simulink model "Propeller"  (R2021a)
settings: Solver=VariableStepAuto  StartTime=0.0  StopTime=10.0  RelTol=1e-3
values from neighbouring files (symbols this model uses):
  param = struct()    [parameters.m]
libraries: vrlib x1
settings Model: Creator=PC  LastModifiedBy=PC

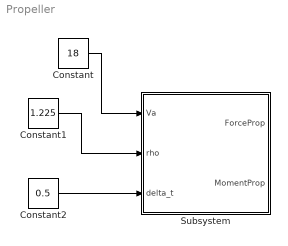
== system Propeller ==
  Constant : Constant  Value=18
  Constant1 : Constant  Value=1.225
  Constant2 : Constant  Value=0.5
  Subsystem : Subsystem
  wires:
  Constant/1 -> Subsystem/1(Va)
  Constant1/1 -> Subsystem/2(rho)
  Constant2/1 -> Subsystem/3(delta_t)

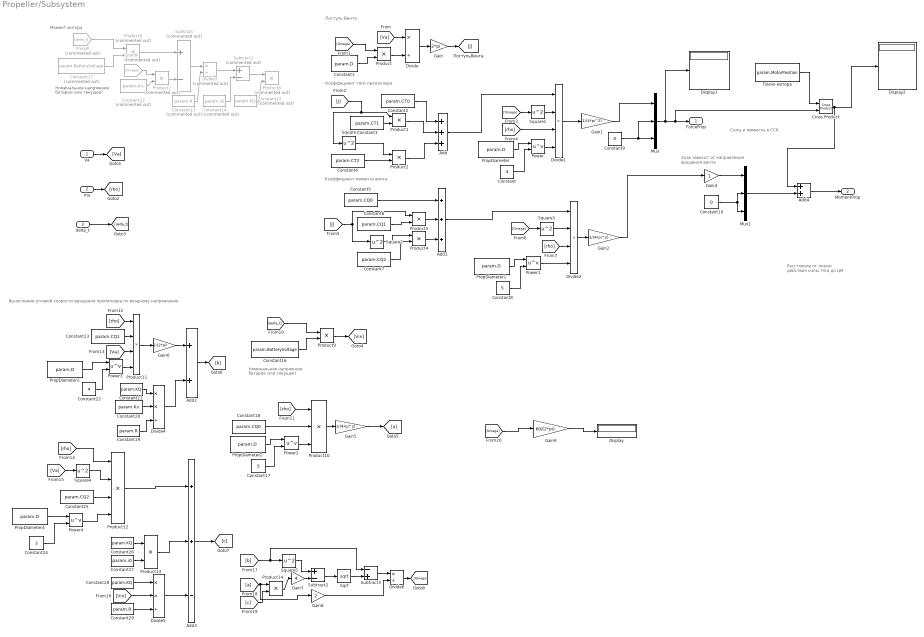
== system Propeller/Subsystem ==
  note: Вычисление угловой скорости вращения пропеллера по входному напряжению
  note: Момент мотора
  note: Номинальное напряжние
      | батарии или текущее?
  note: Знак зависит от направления
      | вращения винта
  note: Силы и моменты в ССК
  note: Расстояние от линии
      | действия силы тяги до ЦМ
  note: Коэффициент момента винта
  note: Коэффициент тяги пропеллера
  note: Поступь Винта
  note: Номинальное напряжние
      | батарии или текущее?
  Va : Inport
  rho : Inport  Port=2
  delta_t : Inport  Port=3
  Add : Sum  Inputs=+++
  Add1 : Sum  Inputs=+++
  Add2 : Sum
  Add3 : Sum  Inputs=++-
  Add4 : Sum
  Constant : Constant  Value=4
  Constant1 : Constant  Value=param.D
  Constant10 : Constant  Value=0
  Constant11 : Constant  Commented=on  Value=param.BatteryVoltage
  Constant12 : Constant  Commented=on  Value=param.Kv
  Constant13 : Constant  Commented=on  Value=param.R
  Constant14 : Constant  Commented=on  Value=param.i0
  Constant15 : Constant  Commented=on  Value=param.KQ
  Constant16 : Constant  Value=param.BatteryVoltage
  Constant17 : Constant  Value=5
  Constant18 : Constant  Value=param.CQ0
  Constant19 : Constant  Value=param.R
  Constant2 : Constant  Value=param.CT0
  Constant20 : Constant  Value=param.Kv
  Constant21 : Constant  Value=param.KQ
  Constant22 : Constant  Value=4
  Constant23 : Constant  Value=param.CQ1
  Constant24 : Constant  Value=3
  Constant25 : Constant  Value=param.CQ2
  Constant26 : Constant  Value=param.KQ
  Constant27 : Constant  Value=param.i0
  Constant28 : Constant  Value=param.KQ
  Constant29 : Constant  Value=param.R
  Constant3 : Constant  Value=param.CT1
  Constant4 : Constant  Value=param.CT2
  Constant5 : Constant  Value=param.CQ0
  Constant6 : Constant  Value=param.CQ1
  Constant7 : Constant  Value=param.CQ2
  Constant8 : Constant  Value=5
  Constant9 : Constant  Value=0
  Cross Product : vrlib/Utilities/Cross Product
  Display : Display
  Display1 : Display
  Display2 : Display
  Divide : Product  Inputs=*/
  Divide1 : Product  Inputs=****
  Divide2 : Product  Inputs=****
  Divide3 : Product  Commented=on  Inputs=*/
  Divide4 : Product  Inputs=**/
  Divide5 : Product  Inputs=**/
  Divide6 : Product  Inputs=*/
  From8 : From  Commented=on  GotoTag=delta_t
  From9 : From  Commented=on  GotoTag=Omega
  Gain : Gain  Gain=2*pi
  Gain1 : Gain  Gain=1/(4*pi^2)
  Gain2 : Gain  Gain=1/(4*pi^2)
  Gain4 : Gain
  Gain5 : Gain  Gain=1/(4*pi^2)
  Gain6 : Gain  Gain=1/(2*pi)
  Gain7 : Gain  Gain=4
  Gain8 : Gain  Gain=2
  Gain9 : Gain  Gain=60/(2*pi)
  Mux : Mux  Inputs=3
  Mux1 : Mux  Inputs=3
  Power{,1..4} (5 alike) : Math  Operator=pow  SaturateOnIntegerOverflow=on
  Product{,1..4,9,13..14} (8 alike) : Product
  Product10 : Product  Inputs=3
  Product11 : Product  Inputs=4
  Product12 : Product  Inputs=4
  Product6 : Product  Commented=on
  Product7 : Product  Commented=on
  Product8 : Product  Commented=on
  PropDiameter{,1..4} (5 alike) : Constant  Value=param.D
  Sqrt : Sqrt  SaturateOnIntegerOverflow=on
  Square{,1..5} (6 alike) : Math  Operator=square  SaturateOnIntegerOverflow=on
  Subtract : Sum  Commented=on  Inputs=+-
  Subtract1 : Sum  Commented=on  Inputs=+-
  Subtract2 : Sum  Inputs=+-
  Subtract3 : Sum  Inputs=-+
  Плечо мотора : Constant  Value=param.MotorPosition
  ForceProp : Outport
  MomentProp : Outport  Port=2
  wires:
  PropDiameter/1 -> Power/1
  Constant/1 -> Power/2
  Va/1 -> [Va]
  Divide/1 -> Gain/1
  Gain/1 -> [J]
  [Va] -> Divide/1
  Product/1 -> Divide/2
  [Omega] -> Product/1
  Constant1/1 -> Product/2
  rho/1 -> [rho]
  Product1/1 -> Add/2
  Product2/1 -> Add/3
  Constant2/1 -> Add/1
  Constant3/1 -> Product1/2
  Constant4/1 -> Product2/2
  [J] -> Product1/1, Square/1
  Square/1 -> Product2/1
  Divide1/1 -> Gain1/1
  Add/1 -> Divide1/1
  [Omega] -> Square1/1
  Square1/1 -> Divide1/2
  [rho] -> Divide1/3
  Power/1 -> Divide1/4
  Constant5/1 -> Add1/1
  Product3/1 -> Add1/2
  [J] -> Product3/1, Square2/1
  Constant6/1 -> Product3/2
  Product4/1 -> Add1/3
  Constant7/1 -> Product4/2
  Square2/1 -> Product4/1
  Add1/1 -> Divide2/1
  [Omega] -> Square3/1
  Square3/1 -> Divide2/2
  Divide2/1 -> Gain2/1
  [rho] -> Divide2/3
  Constant8/1 -> Power1/2
  PropDiameter1/1 -> Power1/1
  Power1/1 -> Divide2/4
  Mux/1 -> Cross Product/2, ForceProp/1, Display1/1
  Gain1/1 -> Mux/1
  Constant9/1 -> Mux/3, Mux/2
  Gain2/1 -> Gain4/1
  Mux1/1 -> Add4/2
  Плечо мотора/1 -> Cross Product/1
  Constant10/1 -> Mux1/3, Mux1/2
  Gain4/1 -> Mux1/1
  delta_t/1 -> [delta_t]
  Constant11/1 -> Product6/2
  From8/1 -> Product6/1
  Product6/1 -> Subtract/1
  Product7/1 -> Subtract/2
  Constant12/1 -> Product7/2
  From9/1 -> Product7/1
  Subtract/1 -> Divide3/1
  Constant13/1 -> Divide3/2
  Divide3/1 -> Subtract1/1
  Constant14/1 -> Subtract1/2
  Subtract1/1 -> Product8/1
  Constant15/1 -> Product8/2
  Constant16/1 -> Product9/2
  [delta_t] -> Product9/1
  Product9/1 -> [Vin]
  [rho] -> Product10/1
  Constant17/1 -> Power2/2
  PropDiameter2/1 -> Power2/1
  Power2/1 -> Product10/3
  Constant18/1 -> Product10/2
  Product10/1 -> Gain5/1
  Gain5/1 -> [a]
  Divide4/1 -> Add2/2
  Constant19/1 -> Divide4/3
  Constant20/1 -> Divide4/2
  Constant21/1 -> Divide4/1
  Product11/1 -> Gain6/1
  Gain6/1 -> Add2/1
  [rho] -> Product11/1
  Constant22/1 -> Power3/2
  PropDiameter3/1 -> Power3/1
  Power3/1 -> Product11/4
  Constant23/1 -> Product11/2
  [Va] -> Product11/3
  Add2/1 -> [b]
  Product12/1 -> Add3/1
  [rho] -> Product12/1
  Constant24/1 -> Power4/2
  PropDiameter4/1 -> Power4/1
  Power4/1 -> Product12/4
  [Va] -> Square4/1
  Square4/1 -> Product12/2
  Constant25/1 -> Product12/3
  Product13/1 -> Add3/2
  Constant26/1 -> Product13/1
  Constant27/1 -> Product13/2
  Divide5/1 -> Add3/3
  Constant28/1 -> Divide5/1
  Constant29/1 -> Divide5/3
  [Vin] -> Divide5/2
  Add3/1 -> [c]
  [b] -> Subtract3/1, Square5/1
  Square5/1 -> Subtract2/1
  [a] -> Product14/1, Gain8/1
  [c] -> Product14/2
  Product14/1 -> Gain7/1
  Subtract2/1 -> Sqrt/1
  Sqrt/1 -> Subtract3/2
  Gain7/1 -> Subtract2/2
  Subtract3/1 -> Divide6/1
  Gain8/1 -> Divide6/2
  Divide6/1 -> [Omega]
  [Omega] -> Gain9/1
  Gain9/1 -> Display/1
  Cross Product/1 -> Add4/1, Display2/1
  Add4/1 -> MomentProp/1
